simulink model "ProofofConceptProblem"  (R2024b)
settings: Solver=ode45  StartTime=0.0  StopTime=25.0  MaxStep=1e-3  RelTol=1e-6  AbsTol=1e-8
values from neighbouring files (symbols this model uses):
  D = qbar*p.S*CD    [uav_longitudinal_dyn.m]
undefined symbols (not defined in the file or in its folder): A, B, C, kd, ki, kp, N
libraries: slpidlib x1
settings Model: Creator=palla  LastModifiedBy=palla
settings DataIOCC: SaveOutput=off  SaveTime=off  ReturnWorkspaceOutputs=off

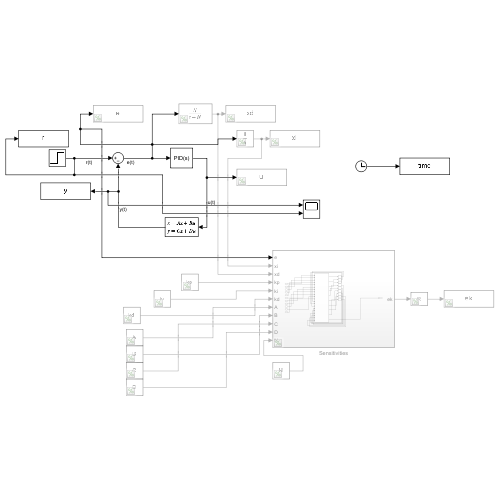
[thumbnail: Simulink's stored preview of the top-level diagram]
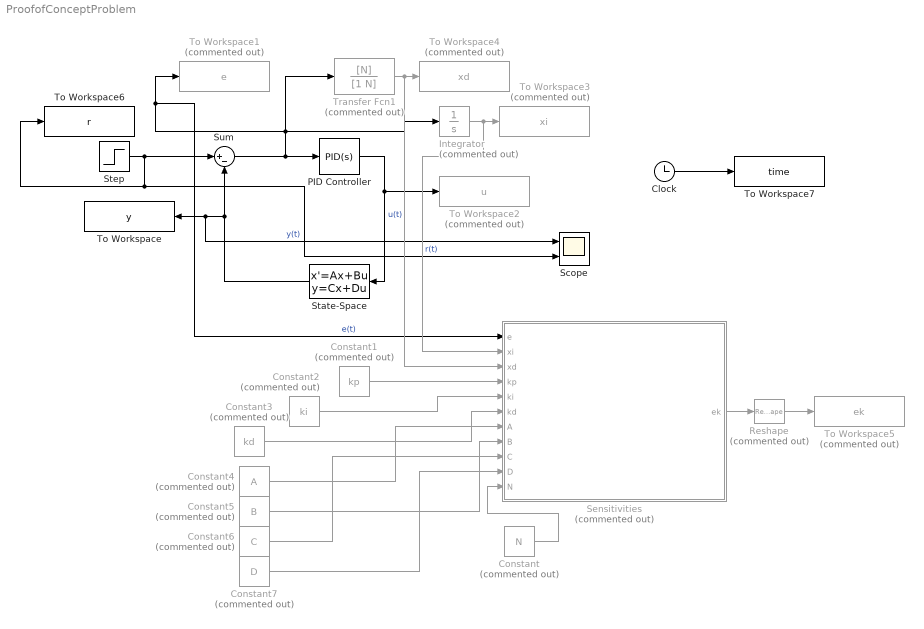
== system ProofofConceptProblem ==
  Clock : Clock
  Constant : Constant  Commented=on  Value=N
  Constant1 : Constant  Commented=on  Value=kp
  Constant2 : Constant  Commented=on  Value=ki
  Constant3 : Constant  Commented=on  Value=kd
  Constant4 : Constant  Commented=on  Value=A  VectorParams1D=off  SampleTime=-1
  Constant5 : Constant  Commented=on  Value=B  VectorParams1D=off  SampleTime=-1
  Constant6 : Constant  Commented=on  Value=C  VectorParams1D=off  SampleTime=-1
  Constant7 : Constant  Commented=on  Value=D  VectorParams1D=off  SampleTime=-1
  Integrator : Integrator  Commented=on
  PID Controller : slpidlib/PID Controller  Controller=PID  Form=Parallel  TimeDomain=Continuous-time  UseExternalTs=off  SampleTime=-1  IntegratorMethod=Forward Euler  FilterMethod=Forward Euler  ControllerParametersSource=internal  P=kp  I=ki  UseKiTs=off  D=kd  UseExternalDerivativeSource=off  N=N  UseFilter=on  TunerSelectOption=Transfer Function Based (PID Tuner App)  InitialConditionSource=internal  InitialConditionForIntegrator=0  InitialConditionForFilter=0  DifferentiatorICPrevScaledInput=0  ExternalReset=none  TrackingMode=off  Kt=1  LimitOutput=off  SatLimitsSource=internal  UpperSaturationLimit=inf  LowerSaturationLimit=-inf  LinearizeAsGain=on  AntiWindupMode=none  Kb=1  LimitIntegrator=off  UpperIntegratorSaturationLimit=inf  LowerIntegratorSaturationLimit=-inf  POutMin=[]  POutMax=[]  IOutMin=[]  IOutMax=[]  DOutMin=[]  DOutMax=[]  NOutMin=[]  NOutMax=[]  SumOutMin=[]  SumOutMax=[]  SaturationOutMin=[]  SaturationOutMax=[]  PParamMin=[]  PParamMax=[]  IParamMin=[]  IParamMax=[]  DParamMin=[]  DParamMax=[]  NParamMin=[]  NParamMax=[]  KbParamMin=[]  KbParamMax=[]  KtParamMin=[]  KtParamMax=[]  KbOutMin=[]  KbOutMax=[]  KtOutMin=[]  KtOutMax=[]  IntegratorOutMin=[]  IntegratorOutMax=[]  FilterOutMin=[]  FilterOutMax=[]  SumI1OutMin=[]  SumI1OutMax=[]  SumI2OutMin=[]  SumI2OutMax=[]  SumI3OutMin=[]  SumI3OutMax=[]  SumI4OutMin=[]  SumI4OutMax=[]  SumDOutMin=[]  SumDOutMax=[]  DifferentiatorOutMin=[]  DifferentiatorOutMax=[]  FilterDiffOutCoefMin=[]  FilterDiffOutCoefMax=[]  ReciprocalOutMin=[]  ReciprocalOutMax=[]  SumDenOutMin=[]  SumDenOutMax=[]  SumNumOutMin=[]  SumNumOutMax=[]  DivideOutMin=[]  DivideOutMax=[]  UdiffTsProdOutMin=[]  UdiffTsProdOutMax=[]  NTsProdOutMin=[]  NTsProdOutMax=[]  UintegralTsProdOutMin=[]  UintegralTsProdOutMax=[]  UngainTsProdOutMin=[]  UngainTsProdOutMax=[]  ClampingZeroOutDataTypeStr=Inherit: Inherit via back propagation  ClampingZeroOutMin=[]  ClampingZeroOutMax=[]  FilterDenConstantOutDataTypeStr=Inherit: Inherit via back propagation  FilterDenConstantOutMin=[]  FilterDenConstantOutMax=[]  PCopyOutDataTypeStr=Inherit: Inherit via back propagation  PCopyOutMin=[]  PCopyOutMax=[]  NCopyOutDataTypeStr=Inherit: Inherit via back propagation  NCopyOutMin=[]  NCopyOutMax=[]  IntegratorContinuousStateAttributes=''  IntegratorStateMustResolveToSignalObject=off  IntegratorRTWStateStorageClass=Auto  FilterContinuousStateAttributes=''  FilterStateMustResolveToSignalObject=off  FilterRTWStateStorageClass=Auto  ParallelPVariant=InternalParameters  IdealPVariant=Disabled  IVariant=InternalParameters  DVariant=InternalParameters  IntegratorVariant=Continuous  SatVariant=Disabled  AWVariant=Passthrough  PCopyVariant=Disabled  TRVariant=Disabled  FdbkBlocksVariant=Forward  IdealPFdbkVariant=Disabled  SatFdbkVariant=Disabled  DerivativeFilterVariant=ContFilter  NVariant=InternalParameters  NCopyVariant=Disabled  FilterICVariant=InternalICsFilter  IntegratorICVariant=InternalICs  ExternalResetVariant=Disabled  TRSumVariant=Passthrough  SumFdbkVariant=Disabled  SumVariant=Sum_PID  TsampFilterVariant=InternalTs  TsampNgainVariant=Passthrough  TsampIntegralVariant=Disabled_SignalSpec  ExternalSaturationOutDataTypeStr=Inherit: Same as second input  DerivativeSourceVariant=ErrorSignal  PreIntVariant=InternalPreInt
  Reshape : Reshape  Commented=on  OutputDimensionality=Customize  OutputDimensions=[3,1]
  Scope : Scope  NumInputPorts=2
  Sensitivities : Subsystem  Commented=on
  State-Space : StateSpace  A=[-2,-6;1,0]  B=[1;0]  C=[1,1]  D=[0]  InitialCondition=0
  Step : Step  Time=0  SampleTime=0
  Sum : Sum  Inputs=|+-
  To Workspace : ToWorkspace  VariableName=y  SampleTime=-1
      settings: Save2DSignal=2-D array (concatenate along first dimension)
  To Workspace1 : ToWorkspace  Commented=on  VariableName=e  SampleTime=-1
      settings: Save2DSignal=2-D array (concatenate along first dimension)
  To Workspace2 : ToWorkspace  Commented=on  VariableName=u  SampleTime=-1
      settings: Save2DSignal=2-D array (concatenate along first dimension)
  To Workspace3 : ToWorkspace  Commented=on  VariableName=xi  SampleTime=-1
      settings: Save2DSignal=2-D array (concatenate along first dimension)
  To Workspace4 : ToWorkspace  Commented=on  VariableName=xd  SampleTime=-1
      settings: Save2DSignal=2-D array (concatenate along first dimension)
  To Workspace5 : ToWorkspace  Commented=on  VariableName=ek  SampleTime=-1
      settings: Save2DSignal=2-D array (concatenate along first dimension)
  To Workspace6 : ToWorkspace  VariableName=r  SampleTime=-1
      settings: Save2DSignal=2-D array (concatenate along first dimension)
  To Workspace7 : ToWorkspace  VariableName=time  SampleTime=-1
      settings: Save2DSignal=2-D array (concatenate along first dimension)
  Transfer Fcn1 : TransferFcn  Commented=on  Numerator=[N]  Denominator=[1 N]
  wires:
  Step/1 -> Scope/2, To Workspace6/1, Sum/1  "r(t)"
  Sum/1 -> Sensitivities/1(e), To Workspace1/1, Transfer Fcn1/1, Integrator/1, PID Controller/1  "e(t)"
  PID Controller/1 -> State-Space/1, To Workspace2/1  "u(t)"
  State-Space/1 -> Sum/2, Scope/1, To Workspace/1  "y(t)"
  Integrator/1 -> Sensitivities/2(xi), To Workspace3/1
  Transfer Fcn1/1 -> Sensitivities/3(xd), To Workspace4/1
  Constant/1 -> Sensitivities/11(N)
  Sensitivities/1(ek) -> Reshape/1
  Constant1/1 -> Sensitivities/4(kp)
  Constant2/1 -> Sensitivities/5(ki)
  Constant3/1 -> Sensitivities/6(kd)
  Constant4/1 -> Sensitivities/7(A)
  Constant5/1 -> Sensitivities/8(B)
  Constant6/1 -> Sensitivities/9(C)
  Constant7/1 -> Sensitivities/10(D)
  Reshape/1 -> To Workspace5/1
  Clock/1 -> To Workspace7/1

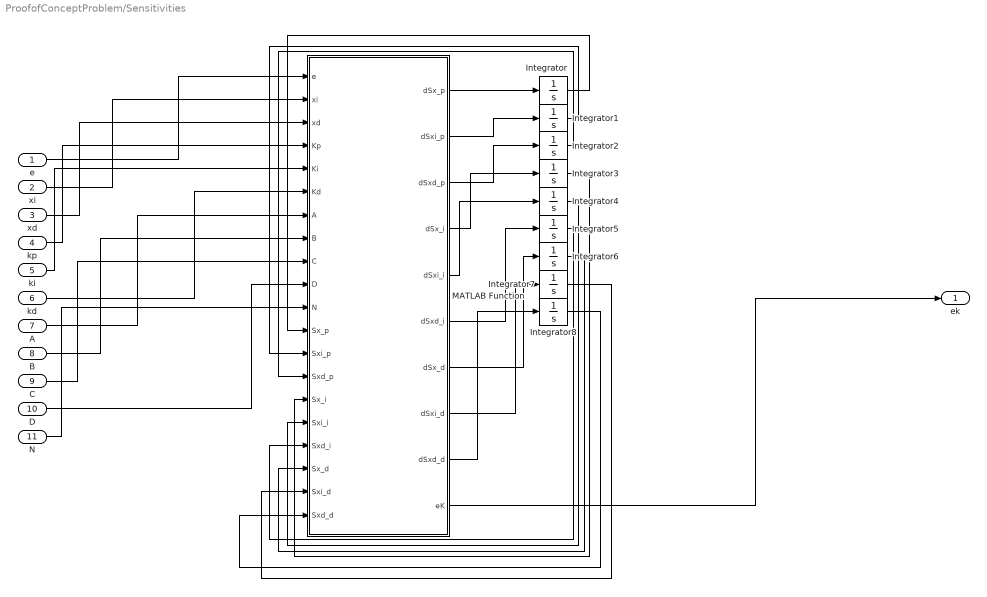
== system ProofofConceptProblem/Sensitivities ==
  e : Inport
  xi : Inport  Port=2
  xd : Inport  Port=3
  kp : Inport  Port=4
  ki : Inport  Port=5
  kd : Inport  Port=6
  A : Inport  Port=7
  B : Inport  Port=8
  C : Inport  Port=9
  D : Inport  Port=10
  N : Inport  Port=11
  Integrator : Integrator  InitialCondition=[0; 0]
  Integrator{1..2,4..5,7..8} (6 alike) : Integrator
  Integrator3 : Integrator  InitialCondition=[0; 0]
  Integrator6 : Integrator  InitialCondition=[0; 0]
  MATLAB Function : MATLAB Function  TreatAsAtomicUnit=on
  ek : Outport
  wires:
  e/1 -> MATLAB Function/1(e)
  xi/1 -> MATLAB Function/2(xi)
  xd/1 -> MATLAB Function/3(xd)
  kp/1 -> MATLAB Function/4(Kp)
  ki/1 -> MATLAB Function/5(Ki)
  kd/1 -> MATLAB Function/6(Kd)
  A/1 -> MATLAB Function/7(A)
  B/1 -> MATLAB Function/8(B)
  C/1 -> MATLAB Function/9(C)
  D/1 -> MATLAB Function/10(D)
  N/1 -> MATLAB Function/11(N)
  MATLAB Function/1(dSx_p) -> Integrator/1
  MATLAB Function/2(dSxi_p) -> Integrator1/1
  MATLAB Function/3(dSxd_p) -> Integrator2/1
  MATLAB Function/4(dSx_i) -> Integrator3/1
  MATLAB Function/5(dSxi_i) -> Integrator4/1
  MATLAB Function/6(dSxd_i) -> Integrator5/1
  MATLAB Function/7(dSx_d) -> Integrator6/1
  MATLAB Function/8(dSxi_d) -> Integrator7/1
  MATLAB Function/9(dSxd_d) -> Integrator8/1
  MATLAB Function/10(eK) -> ek/1
  Integrator/1 -> MATLAB Function/12(Sx_p)
  Integrator1/1 -> MATLAB Function/13(Sxi_p)
  Integrator2/1 -> MATLAB Function/14(Sxd_p)
  Integrator3/1 -> MATLAB Function/15(Sx_i)
  Integrator4/1 -> MATLAB Function/16(Sxi_i)
  Integrator5/1 -> MATLAB Function/17(Sxd_i)
  Integrator6/1 -> MATLAB Function/18(Sx_d)
  Integrator7/1 -> MATLAB Function/19(Sxi_d)
  Integrator8/1 -> MATLAB Function/20(Sxd_d)

== matlab function ProofofConceptProblem/Sensitivities/MATLAB Function ==
  data: e input; dSx_p output; xi input; xd input; Kp input; Ki input; Kd input; A input; B input; C input; D input; N input; Sx_p input; Sxi_p input; Sxd_p input; Sx_i input; Sxi_i input; Sxd_i input; Sx_d input; Sxi_d input; Sxd_d input; dSxi_p output; dSxd_p output; dSx_i output; dSxi_i output; dSxd_i output; dSx_d output; dSxi_d output; dSxd_d output; eK output
function [dSx_p,dSxi_p,dSxd_p, dSx_i,dSxi_i,dSxd_i, dSx_d,dSxi_d,dSxd_d, eK] = ...
         pid_sens_rhs(e, xi, xd, Kp, Ki, Kd, A, B, C, D, N, ...
                      Sx_p, Sxi_p, Sxd_p, Sx_i, Sxi_i, Sxd_i, Sx_d, Sxi_d, Sxd_d)
%#codegen
% PID with filtered D on error: u = Kp*e + Ki*xi + Kd*N*(e - xd)
% Plant D=0 for your model.

ex  = -C;          % de/dx
ux  = Kp*ex;       % du/dx
uxi = Ki;          % du/dxi
uxd = -Kd*N;       % du/dxd
u_Kp = e;          u_Ki = xi;          u_Kd = N*(e - xd);

phi = @(Sx,Sxi,Sxd) ux*Sx + uxi*Sxi + uxd*Sxd;  % scalar
psi = @(Sx)          ex*Sx;                     % since D=0

% --- Kp channel
phi_p  = phi(Sx_p,Sxi_p,Sxd_p);  psi_p  = psi(Sx_p);
dSx_p  = A*Sx_p + B*(phi_p + u_Kp);
dSxi_p = psi_p;
dSxd_p = -N*Sxd_p + N*psi_p;

% --- Ki channel
phi_i  = phi(Sx_i,Sxi_i,Sxd_i);  psi_i  = psi(Sx_i);
dSx_i  = A*Sx_i + B*(phi_i + u_Ki);
dSxi_i = psi_i;
dSxd_i = -N*Sxd_i + N*psi_i;

% --- Kd channel
phi_d  = phi(Sx_d,Sxi_d,Sxd_d);  psi_d  = psi(Sx_d);
dSx_d  = A*Sx_d + B*(phi_d + u_Kd);
dSxi_d = psi_d;
dSxd_d = -N*Sxd_d + N*psi_d;

% ∂e/∂K = -∂y/∂K, with ∂y/∂K = C*Sx_j  (D=0)
% make it column: 3x1  -> logs as Nx3
eK = -[C*Sx_p; C*Sx_i; C*Sx_d];
